simulink model "amk_sim_model"  (R2022b)
settings: Solver=FixedStepAuto  StartTime=0.0  StopTime=4  FixedStep=1e-6  MaxStep=1e-5  MinStep=1e-6  RelTol=1e-3
values from neighbouring files (symbols this model uses):
  a_fw = log(9)/trfw    [amk_sim.m]    (also in amk_sim_2.m)
  ac = log(9)/tr    [amk_sim.m]    (also in amk_sim_2.m)
  ar_max = 1500    [amk_sim_2.m]
  as = log(9)/trs    [amk_sim.m]    (also in amk_sim_2.m)
  ba = 2*k^2*(as*J - 0)/(np^2*psi)    [amk_sim.m]    (also in amk_sim_2.m = 2*k^2*(as*J - bm)/(np^2*psi))
  bm = 0.02    [amk_sim.m]    (also in amk_sim_2.m = 0.008)
  I_base = 85.7    [amk_sim.m]    (also in amk_sim_2.m)
  I_max = 85.7    [amk_sim.m]    (also in amk_sim_2.m)
  Icon = 33.5    [amk_sim.m]    (also in amk_sim_2.m)
  Imax_interval = 1.24    [amk_sim.m]    (also in amk_sim_2.m = 5)
  Ipeak = 85.7    [amk_sim.m]    (also in amk_sim_2.m = 87.5)
  J = 2.5*(2.74e-4)    (= 0.000685)    [amk_sim.m]    (also in amk_sim_2.m = 0.000528)
  k = 1    [amk_sim.m]    (also in amk_sim_2.m)
  ki_ar = 0.2    [amk_sim_2.m]
  ki_s = 2*k^2*as^2*J/(np^2*psi)    [amk_sim.m]    (also in amk_sim_2.m)
  kp_ar = 1e-5    (= 1e-05)    [amk_sim_2.m]
  kp_s = 2*k^2*as*J/(np^2*psi)    [amk_sim.m]    (also in amk_sim_2.m)
  Ld = Ldm    (= 0.0004)    [amk_sim.m]    (also in amk_sim_2.m = 0.00012)
  Lq = Lqm    (= 0.00052)    [amk_sim.m]    (also in amk_sim_2.m = 0.00024)
  max_temp = 140    [amk_sim.m]    (also in amk_sim_2.m)
  np = 5    [amk_sim.m]    (also in amk_sim_2.m)
  Peak_power = 45000    [amk_sim.m]    (also in amk_sim_2.m = 50000)
  Peak_regen = -15000    [amk_sim.m]    (also in amk_sim_2.m = -1500000)
  psi = 0.047    [amk_sim.m]    (also in amk_sim_2.m = 0.05077789)
  rpm_nom = 20000    [amk_sim.m]    (also in amk_sim_2.m = 12000)
  Rs = 202.5e-3    (= 0.2025)    [amk_sim.m]    (also in amk_sim_2.m)
  sample_time = 1e-4    (= 0.0001)    [amk_sim.m]    (also in amk_sim_2.m = 1e-06)
  temp_threshold = 100    [amk_sim.m]    (also in amk_sim_2.m)
  u_dc = 550    [amk_sim.m]    (also in amk_sim_2.m)
  u_nom = u_dc*k    (= 550)    [amk_sim.m]    (also in amk_sim_2.m)
undefined symbols (not defined in the file or in its folder): sigbuilder_block
libraries: simulink x3
(part 2 of 5)

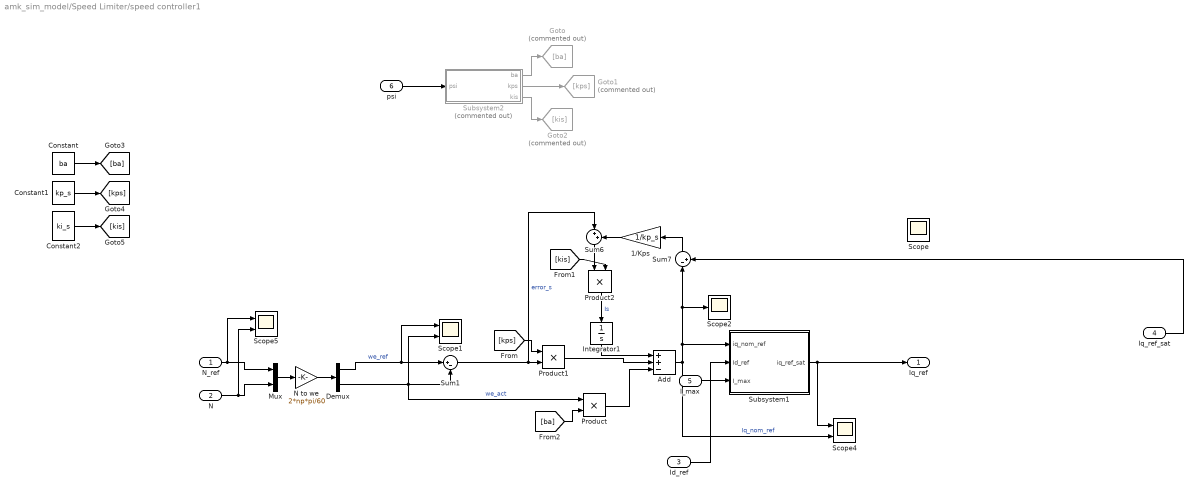
== system amk_sim_model/Speed Limiter/speed controller1 ==
  N_ref : Inport
  N : Inport  Port=2
  Id_ref : Inport  Port=3
  Iq_ref_sat : Inport  Port=4
  I_max : Inport  Port=5
  psi : Inport  Port=6
  1/Kps : Gain  Gain=1/kp_s
  Add : Sum  Inputs=++-
  Constant : Constant  Value=ba
  Constant1 : Constant  Value=kp_s
  Constant2 : Constant  Value=ki_s
  Demux : Demux  Outputs=2
  Goto : Goto  Commented=on  GotoTag=ba
  Goto1 : Goto  Commented=on  GotoTag=kps
  Goto2 : Goto  Commented=on  GotoTag=kis
  Integrator1 : Integrator
  Mux : Mux  Inputs=2
  N to we : Gain  Gain=2*np*pi/60
  Product : Product
  Product1 : Product
  Product2 : Product
  Scope : Scope
  Scope1 : Scope  NumInputPorts=2
  Scope2 : Scope
  Scope4 : Scope  NumInputPorts=2
  Scope5 : Scope  NumInputPorts=2
  Subsystem1 : Subsystem
  Subsystem2 : Subsystem  Commented=on
  Sum1 : Sum  Inputs=|+-
  Sum6 : Sum  Inputs=|++
  Sum7 : Sum  Inputs=|-+
  Iq_ref : Outport
  wires:
  [kis] -> Product2/2
  [kps] -> Product1/1
  Subsystem2/3(kis) -> Goto2/1
  Subsystem2/2(kps) -> Goto1/1
  Subsystem2/1(ba) -> Goto/1
  psi/1 -> Subsystem2/1(psi)
  I_max/1 -> Subsystem1/3(I_max)
  Iq_ref_sat/1 -> Sum7/2
  Id_ref/1 -> Subsystem1/2(Id_ref)
  Integrator1/1 -> Add/1
  N to we/1 -> Demux/1
  Mux/1 -> N to we/1
  Subsystem1/1(iq_ref_sat) -> Iq_ref/1, Scope4/1
  Sum6/1 -> Product2/1
  Demux/2 -> Scope1/2, Sum1/2, Product/1  "we_act"
  Demux/1 -> Sum1/1, Scope1/1  "we_ref"
  Product/1 -> Add/3
  Product2/1 -> Integrator1/1  "Is"
  [ba] -> Product/2
  N/1 -> Mux/2, Scope5/2
  N_ref/1 -> Mux/1, Scope5/1
  Sum1/1 -> Sum6/1, Product1/2  "error_s"
  1/Kps/1 -> Sum6/2
  Product1/1 -> Add/2
  Add/1 -> Scope4/2, Subsystem1/1(iq_nom_ref), Sum7/1, Scope2/1  "Iq_nom_ref"
  Sum7/1 -> 1/Kps/1
  Constant1/1 -> [kps]
  Constant/1 -> [ba]
  Constant2/1 -> [kis]

== system amk_sim_model/fw controller1/fw gain calculator ==
  we : Inport
  Ld : Inport  Port=2
  Abs : Abs  SaturateOnIntegerOverflow=off
  Constant : Constant  Value=a_fw
  Constant2 : Constant  Value=u_nom
  Constant3 : Constant  Value=rpm_nom
  Divide : Product  Inputs=*/
  Gain : Gain  Gain=2
  Max : MinMax  Function=max  Inputs=2
  N to we : Gain  Gain=2*np*pi/60
  Product : Product  Inputs=3
  Scope1 : Scope  NumInputPorts=2
  Scope2 : Scope
  prevent div by 2 : Subsystem
  Kfw : Outport
  wires:
  Constant3/1 -> N to we/1
  we/1 -> Abs/1
  Abs/1 -> Max/2, Scope1/2  "we"
  Gain/1 -> Product/1
  Constant/1 -> Divide/1
  Max/1 -> Product/3
  Constant2/1 -> Product/2
  Product/1 -> prevent div by 2/1(IN)
  N to we/1 -> Scope1/1, Max/1  "we_max"
  Divide/1 -> Kfw/1, Scope2/1
  Ld/1 -> Gain/1
  prevent div by 2/1(OUT) -> Divide/2

== system amk_sim_model/speed controller/Subsystem1 ==
  iq_nom_ref : Inport
  Id_ref : Inport  Port=2
  I_max : Inport  Port=3
  Add : Sum  Inputs=+-
  Gain : Gain  Gain=-1
  Max : MinMax  Function=max  Inputs=2
  Min : MinMax  Inputs=2
  Scope : Scope
  Square Root : Sqrt
  Square1 : Math  Operator=square
  Square2 : Math  Operator=square
  Unit Delay : UnitDelay  SampleTime=-1  HasFrameUpgradeWarning=on
  iq_ref_sat : Outport
  wires:
  Square2/1 -> Add/1
  iq_nom_ref/1 -> Min/2
  I_max/1 -> Square2/1
  Square1/1 -> Add/2
  Square Root/1 -> Unit Delay/1
  Add/1 -> Square Root/1
  Max/1 -> iq_ref_sat/1
  Gain/1 -> Max/2
  Id_ref/1 -> Square1/1
  Unit Delay/1 -> Min/1, Gain/1, Scope/1
  Min/1 -> Max/1

== system amk_sim_model/speed controller/Subsystem2 ==
  psi : Inport
  Constant : Constant  Value=2*k^2*(as*J)/np^2
  Constant1 : Constant  Value=2*k^2*(as*J)/np^2
  Constant2 : Constant  Value=2*k^2*(as^2*J)/np^2
  Divide : Product  Inputs=*/
  Divide1 : Product  Inputs=*/
  Divide2 : Product  Inputs=*/
  ba : Outport
  kps : Outport  Port=2
  kis : Outport  Port=3
  wires:
  Constant/1 -> Divide/1
  psi/1 -> [psi]
  [psi] -> Divide/2
  [psi] -> Divide1/2
  Constant1/1 -> Divide1/1
  Constant2/1 -> Divide2/1
  [psi] -> Divide2/2
  Divide/1 -> ba/1
  Divide1/1 -> kps/1
  Divide2/1 -> kis/1

== system amk_sim_model/Current Controller/Subsystem/prevent div by 1 ==
  IN : Inport
  Constant : Constant  Value=0.0001
  Switch : Switch  Criteria=u2 > Threshold  Threshold=0.0001  SaturateOnIntegerOverflow=off  InputSameDT=off  OutDataTypeStr=Inherit: Same as first input
  OUT : Outport  VectorParamsAs1DForOutWhenUnconnected=off
  wires:
  IN/1 -> Switch/2, Switch/1
  Switch/1 -> OUT/1
  Constant/1 -> Switch/3

== system amk_sim_model/Current Controller/Subsystem/prevent div by 2 ==
  IN : Inport
  Constant : Constant  Value=0.0001
  Switch : Switch  Criteria=u2 > Threshold  Threshold=0.0001  SaturateOnIntegerOverflow=off  InputSameDT=off  OutDataTypeStr=Inherit: Same as first input
  OUT : Outport  VectorParamsAs1DForOutWhenUnconnected=off
  wires:
  Constant/1 -> Switch/3
  Switch/1 -> OUT/1
  IN/1 -> Switch/1, Switch/2

== system amk_sim_model/Current Controller/Subsystem1/prevent div by 1 ==
  IN : Inport
  Constant : Constant  Value=0.0001
  Switch : Switch  Criteria=u2 > Threshold  Threshold=0.0001  SaturateOnIntegerOverflow=off  InputSameDT=off  OutDataTypeStr=Inherit: Same as first input
  OUT : Outport  VectorParamsAs1DForOutWhenUnconnected=off
  wires:
  IN/1 -> Switch/2, Switch/1
  Switch/1 -> OUT/1
  Constant/1 -> Switch/3

== system amk_sim_model/Current Controller/Subsystem1/prevent div by 2 ==
  IN : Inport
  Constant : Constant  Value=0.0001
  Switch : Switch  Criteria=u2 > Threshold  Threshold=0.0001  SaturateOnIntegerOverflow=off  InputSameDT=off  OutDataTypeStr=Inherit: Same as first input
  OUT : Outport  VectorParamsAs1DForOutWhenUnconnected=off
  wires:
  Constant/1 -> Switch/3
  Switch/1 -> OUT/1
  IN/1 -> Switch/1, Switch/2

== system amk_sim_model/Speed Limiter/speed controller/Subsystem1 ==
  iq_nom_ref : Inport
  Id_ref : Inport  Port=2
  I_max : Inport  Port=3
  Add : Sum  Inputs=+-
  Constant : Constant  Value=0
  Gain : Gain  Gain=-1
  Max : MinMax  Function=max  Inputs=2
  Max1 : MinMax  Function=max  Inputs=2
  Min : MinMax  Inputs=2
  Scope : Scope
  Scope{1..2,4..6} (5 alike) : Scope  NumInputPorts=2
  Scope3 : Scope  NumInputPorts=3
  Square Root : Sqrt
  Square1 : Math  Operator=square
  Square2 : Math  Operator=square
  Unit Delay : UnitDelay  SampleTime=-1  HasFrameUpgradeWarning=on
  iq_ref_sat : Outport
  wires:
  Square2/1 -> Add/1
  iq_nom_ref/1 -> Scope3/2, Min/2
  I_max/1 -> Scope4/2, Scope1/1, Square2/1
  Square1/1 -> Add/2
  Square Root/1 -> Scope1/2, Unit Delay/1
  Add/1 -> Max1/1
  Max/1 -> Scope2/1, iq_ref_sat/1
  Gain/1 -> Max/2
  Id_ref/1 -> Square1/1
  Unit Delay/1 -> Scope5/1, Scope3/1, Min/1, Gain/1, Scope/1
  Min/1 -> Scope3/3, Max/1
  Max1/1 -> Scope6/1, Square Root/1
  Constant/1 -> Max1/2

== system amk_sim_model/Speed Limiter/speed controller/Subsystem2 ==
  psi : Inport
  Constant : Constant  Value=2*k^2*(as*J)/np^2
  Constant1 : Constant  Value=2*k^2*(as*J)/np^2
  Constant2 : Constant  Value=2*k^2*(as^2*J)/np^2
  Divide : Product  Inputs=*/
  Divide1 : Product  Inputs=*/
  Divide2 : Product  Inputs=*/
  ba : Outport
  kps : Outport  Port=2
  kis : Outport  Port=3
  wires:
  Constant/1 -> Divide/1
  psi/1 -> [psi]
  [psi] -> Divide/2
  [psi] -> Divide1/2
  Constant1/1 -> Divide1/1
  Constant2/1 -> Divide2/1
  [psi] -> Divide2/2
  Divide/1 -> ba/1
  Divide1/1 -> kps/1
  Divide2/1 -> kis/1

== system amk_sim_model/Speed Limiter/speed controller1/Subsystem1 ==
  iq_nom_ref : Inport
  Id_ref : Inport  Port=2
  I_max : Inport  Port=3
  Add : Sum  Inputs=+-
  Gain : Gain  Gain=-1
  Max : MinMax  Function=max  Inputs=2
  Min : MinMax  Inputs=2
  Scope : Scope
  Square Root : Sqrt
  Square1 : Math  Operator=square
  Square2 : Math  Operator=square
  Unit Delay : UnitDelay  SampleTime=-1  HasFrameUpgradeWarning=on
  iq_ref_sat : Outport
  wires:
  Id_ref/1 -> Square1/1
  Gain/1 -> Max/2
  Add/1 -> Square Root/1
  Square Root/1 -> Unit Delay/1
  Square1/1 -> Add/2
  I_max/1 -> Square2/1
  iq_nom_ref/1 -> Min/2
  Square2/1 -> Add/1
  Unit Delay/1 -> Min/1, Scope/1, Gain/1
  Min/1 -> Max/1
  Max/1 -> iq_ref_sat/1

== system amk_sim_model/Speed Limiter/speed controller1/Subsystem2 ==
  psi : Inport
  Constant : Constant  Value=2*k^2*(as*J)/np^2
  Constant1 : Constant  Value=2*k^2*(as*J)/np^2
  Constant2 : Constant  Value=2*k^2*(as^2*J)/np^2
  Divide : Product  Inputs=*/
  Divide1 : Product  Inputs=*/
  Divide2 : Product  Inputs=*/
  ba : Outport
  kps : Outport  Port=2
  kis : Outport  Port=3
  wires:
  Divide2/1 -> kis/1
  Divide1/1 -> kps/1
  Divide/1 -> ba/1
  [psi] -> Divide2/2
  Constant2/1 -> Divide2/1
  Constant1/1 -> Divide1/1
  [psi] -> Divide1/2
  [psi] -> Divide/2
  psi/1 -> [psi]
  Constant/1 -> Divide/1

== system amk_sim_model/fw controller1/fw gain calculator/prevent div by 2 ==
  IN : Inport
  Constant : Constant  Value=0.0001
  Switch : Switch  Criteria=u2 > Threshold  Threshold=0.0001  SaturateOnIntegerOverflow=off  InputSameDT=off  OutDataTypeStr=Inherit: Same as first input
  OUT : Outport  VectorParamsAs1DForOutWhenUnconnected=off
  wires:
  Constant/1 -> Switch/3
  Switch/1 -> OUT/1
  IN/1 -> Switch/1, Switch/2

== matlab function amk_sim_model/pm flux est ==
  data: Iq input; psi output
function psi= fcn(Iq)

pm_flux = [47.22932693 47.21431813 47.05146664	46.75587183	46.34316 45.82916949 45.22964911 44.56000026 43.83468728 43.06630479 42.26389314 41.43526414 40.58848093 39.73068354 38.86734457 38.00279887 37.14115431 36.28662807 35.44396164 34.61891364 33.81865599];

Iq_array = [0	4.28660705	8.573214102	12.85982115	17.1464282	21.43303539	25.71964261	30.00624953	34.29285645	38.57946347	42.86607073	47.15267796	51.4392846	55.72589165	60.01249877	64.29910575	68.58571287	72.87231986	77.1589269	81.44553396	85.732141];

if(Iq >= Iq_array(21))
    psi = pm_flux(21)/1000;
else
    i = floor(Iq/4.2866);

    low = Iq_array(i+1);

    precentage = (Iq - low)/Iq_array(2);
    
    psi = (precentage*pm_flux(i+2)+(1-precentage)*pm_flux(i+1))/1000;
end

== matlab function amk_sim_model/I2t/MATLAB Function ==
  data: u input; y output; t input; c input
function y = fcn(u, t, c)
double k;

if (u > c)
    k = 1;
else
    k = -1;
end

if(t < 0.0001)
    k = 1;
end
y = k;
